simulink model "mclosed_loop_sim"  (Simulink 6.3)
settings: Solver=ode23s  SolverMode=SingleTasking  StartTime=0.0  StopTime=10  RelTol=1e-3  AbsTol=1e-6
PreLoadFcn:
  | Kp=0.0614;Ki=0.0723;
undefined symbols (not defined in the file or in its folder): DiscIntNeverNeededParam
settings Model: CovMetricSettings=d  Creator=The MathWorks Inc.  LastModifiedBy=mshakeri  ExtModeTrigMode=oneshot  ExtModeArmWhenConnect=off  ExtModeAutoUpdateStatusClock=off  StrictBusMsg=ErrorLevel1
settings DataIOCC: ExternalInput=[]  InitialState=[]  LimitDataPoints=off  SaveFormat=StructureWithTime  OutputSaveName=yout1
settings OptimizationCC: BooleanDataType=off  InlineParams=on  InlineInvariantSignals=on
settings DebuggingCC: CheckExecutionContextPreStartOutputMsg=on  CheckExecutionContextRuntimeOutputMsg=on  SolverPrmCheckMsg=none  IntegerOverflowMsg=none
settings HardwareCC: TargetUnknown=on

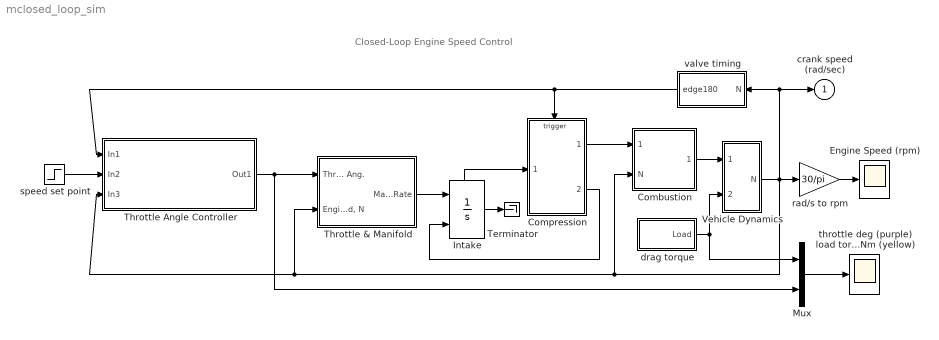
== system mclosed_loop_sim ==
  note: Closed-Loop Engine Speed Control
  Combustion : Subsystem
  Compression : Subsystem  TreatAsAtomicUnit=on
  Engine Speed (rpm) : Scope
      settings: TickLabels=on  YMin=1500  YMax=3500  SaveName=scopeout1
  Intake : Integrator  ExternalReset=either  ShowStatePort=on
  Mux : Mux  Inputs=2
  Terminator : Terminator
  Throttle & Manifold : Subsystem
  Throttle Angle Controller : Subsystem  TreatAsAtomicUnit=on
  Vehicle Dynamics : Subsystem
  drag torque : Subsystem
  rad/s to rpm : Gain  Gain=30/pi  SaturateOnIntegerOverflow=on
  speed set point : Step  Time=5  Before=2000  After=3000  SampleTime=0
  throttle deg (purple) load torque Nm (yellow) : Scope
      settings: TickLabels=on  YMin=5  YMax=30  SaveName=scopeout2
  valve timing : Subsystem  Orientation=left
  crank speed (rad/sec) : Outport  InitialOutput=0
  wires:
  speed set point/1 -> Throttle Angle Controller/2(In2)
  drag torque/1(Load) -> Mux/1, Vehicle Dynamics/2(Tload)
  Throttle Angle Controller/1(Out1) -> Throttle & Manifold/1(Throttle Ang.), Mux/2
  Compression/1(mass(k)) -> Combustion/1(Air Charge)
  Throttle & Manifold/1(Mass Airflow Rate) -> Intake/1
  Intake/1 -> Terminator/1
  Intake/State -> Compression/1(mass(k+1))
  Compression/2(trigger) -> Intake/2
  valve timing/1(edge180) -> Compression/Trigger, Throttle Angle Controller/1(In1)
  Combustion/1(Torque) -> Vehicle Dynamics/1(Teng)
  Vehicle Dynamics/1(N) -> Throttle & Manifold/2("Engine Speed, N"), Throttle Angle Controller/3(In3), Combustion/2(N), valve timing/1(N), crank speed (rad/sec)/1, rad/s to rpm/1
  rad/s to rpm/1 -> Engine Speed (rpm)/1
  Mux/1 -> throttle deg (purple) load torque Nm (yellow)/1

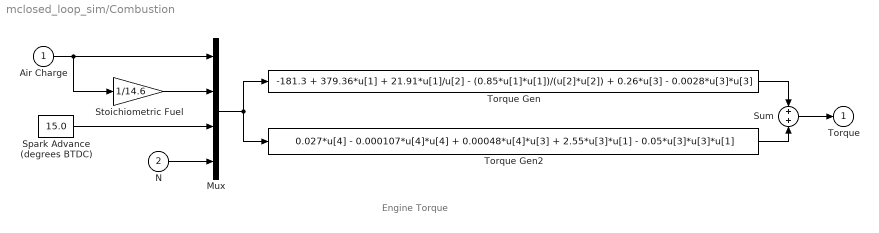
== system mclosed_loop_sim/Combustion ==
  note: Engine Torque
  Air Charge : Inport  Port=1  LatchInput=off
  N : Inport  Port=2  LatchInput=off
  Mux : Mux
  Spark Advance (degrees BTDC) : Constant  Value=15.0
  Stoichiometric Fuel : Gain  Gain=1/14.6  SaturateOnIntegerOverflow=on
  Sum : Sum  SaturateOnIntegerOverflow=on  InputSameDT=on
  Torque Gen : Fcn  Expr=-181.3 + 379.36*u[1] + 21.91*u[1]/u[2] - (0.85*u[1]*u[1])/(u[2]*u[2]) + 0.26*u[3] - 0.0028*u[3]*u[3]
  Torque Gen2 : Fcn  Expr=0.027*u[4] - 0.000107*u[4]*u[4] + 0.00048*u[4]*u[3] + 2.55*u[3]*u[1] - 0.05*u[3]*u[3]*u[1]
  Torque : Outport  InitialOutput=0
  wires:
  Stoichiometric Fuel/1 -> Mux/2
  Spark Advance (degrees BTDC)/1 -> Mux/3
  N/1 -> Mux/4
  Air Charge/1 -> Stoichiometric Fuel/1, Mux/1
  Mux/1 -> Torque Gen/1, Torque Gen2/1
  Torque Gen2/1 -> Sum/2
  Torque Gen/1 -> Sum/1
  Sum/1 -> Torque/1

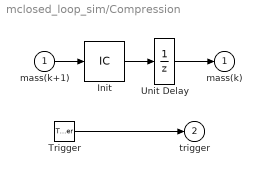
== system mclosed_loop_sim/Compression ==
  mass(k+1) : Inport  Port=1  LatchInput=off
  Trigger : TriggerPort  TriggerType=either  ShowOutputPort=on
  Init : InitialCondition  Value=0.152
  Unit Delay : UnitDelay  X0=0.152  SampleTime=-1
  mass(k) : Outport  InitialOutput=0.152
  trigger : Outport  Port=2  InitialOutput=-1
  wires:
  Init/1 -> Unit Delay/1
  mass(k+1)/1 -> Init/1
  Unit Delay/1 -> mass(k)/1
  Trigger/1 -> trigger/1

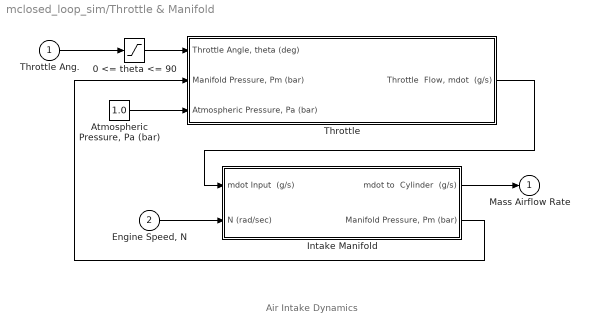
== system mclosed_loop_sim/Throttle & Manifold ==
  note: Air Intake Dynamics
  Throttle Ang. : Inport  Port=1  LatchInput=off
  "Engine Speed, N" : Inport  Port=2  LatchInput=off
  0 <= theta <= 90 : Saturate  UpperLimit=90  LowerLimit=0
  "Atmospheric Pressure, Pa (bar)" : Constant  Value=1.0
  Intake Manifold : Subsystem
  Throttle : Subsystem
  Mass Airflow Rate : Outport  InitialOutput=0
  wires:
  "Atmospheric Pressure, Pa (bar)"/1 -> Throttle/3("Atmospheric Pressure, Pa (bar) ")
  Intake Manifold/1(mdot to  Cylinder  (g/s)) -> Mass Airflow Rate/1
  Intake Manifold/2("Manifold Pressure, Pm (bar)") -> Throttle/2("Manifold Pressure, Pm (bar)")
  "Engine Speed, N"/1 -> Intake Manifold/2(N (rad/sec))
  Throttle/1("Throttle  Flow, mdot  (g/s)") -> Intake Manifold/1(mdot Input  (g/s))
  Throttle Ang./1 -> 0 <= theta <= 90/1
  0 <= theta <= 90/1 -> Throttle/1("Throttle Angle, theta (deg)")

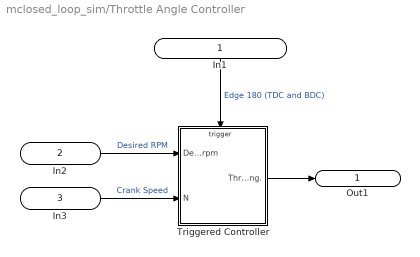
== system mclosed_loop_sim/Throttle Angle Controller ==
  In1 : Inport  Orientation=down  Port=1  LatchInput=off
  In2 : Inport  Port=2  SampleTime=[0 1]  LatchInput=off
  In3 : Inport  Port=3  SampleTime=[0 1]  LatchInput=off
  Triggered Controller : Subsystem  TreatAsAtomicUnit=on
  Out1 : Outport
  wires:
  In1/1 -> Triggered Controller/Trigger  "Edge 180 (TDC and BDC)"
  In3/1 -> Triggered Controller/2(N)  "Crank Speed"
  In2/1 -> Triggered Controller/1(Desired rpm)  "Desired RPM"
  Triggered Controller/1(Throttle Ang.) -> Out1/1

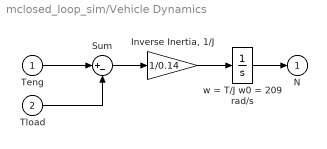
== system mclosed_loop_sim/Vehicle Dynamics ==
  Teng : Inport  Port=1  LatchInput=off
  Tload : Inport  Port=2  LatchInput=off
  "Inverse Inertia, 1/J" : Gain  Gain=1/0.14  SaturateOnIntegerOverflow=on
  Sum : Sum  Inputs=|+-  SaturateOnIntegerOverflow=on  InputSameDT=on
  w = T/J w0 = 209 rad/s : Integrator  InitialCondition=209.48
  N : Outport  InitialOutput=0
  wires:
  "Inverse Inertia, 1/J"/1 -> w = T/J w0 = 209 rad/s/1
  w = T/J w0 = 209 rad/s/1 -> N/1
  Sum/1 -> "Inverse Inertia, 1/J"/1
  Teng/1 -> Sum/1
  Tload/1 -> Sum/2

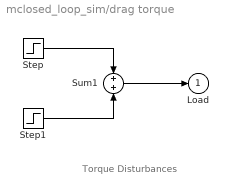
== system mclosed_loop_sim/drag torque ==
  note: Torque Disturbances
  Step : Step  Time=2  Before=25  After=20  SampleTime=0
  Step1 : Step  Time=8  After=5  SampleTime=0
  Sum1 : Sum  SaturateOnIntegerOverflow=on  InputSameDT=on
  Load : Outport  InitialOutput=0
  wires:
  Sum1/1 -> Load/1
  Step/1 -> Sum1/1
  Step1/1 -> Sum1/2

== system mclosed_loop_sim/valve timing ==
  note: Rotational Velocity to Synchronized
      | Discrete Event Conversion
  N : Inport  Orientation=left  Port=1  LatchInput=off
  TDC and BDC detection : Subsystem  Orientation=left
  positive edge to dual edge conversion : Subsystem  Orientation=left  TreatAsAtomicUnit=on
  edge180 : Outport  Orientation=left  InitialOutput=-1
  wires:
  TDC and BDC detection/1(trigger) -> positive edge to dual edge conversion/Trigger
  positive edge to dual edge conversion/1(trigger) -> edge180/1
  N/1 -> TDC and BDC detection/1(N)  "rad/sec"

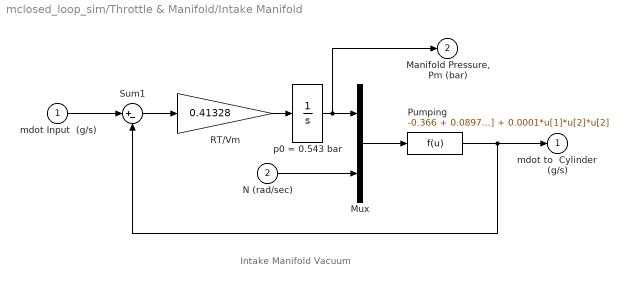
== system mclosed_loop_sim/Throttle & Manifold/Intake Manifold ==
  note: Intake Manifold Vacuum
  mdot Input  (g/s) : Inport  Port=1  LatchInput=off
  N (rad/sec) : Inport  Port=2  LatchInput=off
  Mux : Mux  Inputs=2
  Pumping : Fcn  Expr=-0.366 + 0.08979*u[1]*u[2] - 0.0337*u[2]*u[1]*u[1] + 0.0001*u[1]*u[2]*u[2]
  RT/Vm : Gain  Gain=0.41328  SaturateOnIntegerOverflow=on
  Sum1 : Sum  Inputs=|+-  SaturateOnIntegerOverflow=on  InputSameDT=on
  p0 = 0.543 bar : Integrator  InitialCondition=.543
  mdot to  Cylinder  (g/s) : Outport  InitialOutput=0
  "Manifold Pressure, Pm (bar)" : Outport  Port=2  InitialOutput=0
  wires:
  Pumping/1 -> mdot to  Cylinder  (g/s)/1, Sum1/2
  Sum1/1 -> RT/Vm/1
  p0 = 0.543 bar/1 -> "Manifold Pressure, Pm (bar)"/1, Mux/1
  Mux/1 -> Pumping/1
  N (rad/sec)/1 -> Mux/2
  RT/Vm/1 -> p0 = 0.543 bar/1
  mdot Input  (g/s)/1 -> Sum1/1

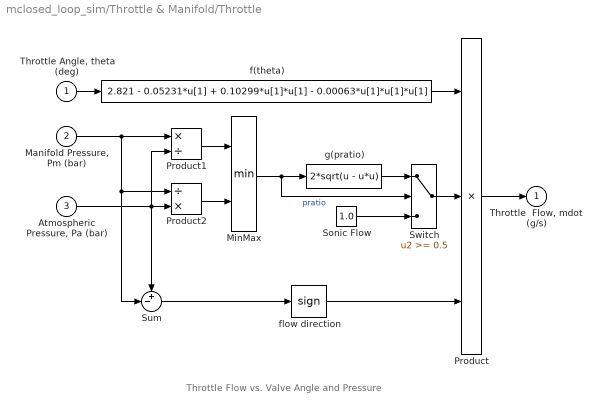
== system mclosed_loop_sim/Throttle & Manifold/Throttle ==
  note: Throttle Flow vs. Valve Angle and Pressure
  "Throttle Angle, theta (deg)" : Inport  Port=1  LatchInput=off
  "Manifold Pressure, Pm (bar)" : Inport  Port=2  LatchInput=off
  "Atmospheric Pressure, Pa (bar) " : Inport  Port=3  LatchInput=off
  MinMax : MinMax  Inputs=2  SaturateOnIntegerOverflow=on  InputSameDT=on
  Product : Product  Inputs=3  SaturateOnIntegerOverflow=on  RndMeth=Zero  InputSameDT=on
  Product1 : Product  Inputs=*/  SaturateOnIntegerOverflow=on  RndMeth=Zero  InputSameDT=on
  Product2 : Product  Inputs=/*  SaturateOnIntegerOverflow=on  RndMeth=Zero  InputSameDT=on
  "Sonic Flow " : Constant  Value=1.0
  Sum : Sum  Inputs=+-|  SaturateOnIntegerOverflow=on  InputSameDT=on
  Switch : Switch  Threshold=0.5  SaturateOnIntegerOverflow=on  InputSameDT=on
  f(theta) : Fcn  Expr=2.821 - 0.05231*u[1] + 0.10299*u[1]*u[1] - 0.00063*u[1]*u[1]*u[1]
  flow direction : Signum
  g(pratio) : Fcn  Expr=2*sqrt(u - u*u)
  "Throttle  Flow, mdot  (g/s)" : Outport  InitialOutput=0
  wires:
  f(theta)/1 -> Product/1
  Product/1 -> "Throttle  Flow, mdot  (g/s)"/1
  "Throttle Angle, theta (deg)"/1 -> f(theta)/1
  MinMax/1 -> g(pratio)/1, Switch/2  "pratio"
  Sum/1 -> flow direction/1
  flow direction/1 -> Product/3
  Switch/1 -> Product/2
  "Sonic Flow "/1 -> Switch/3
  g(pratio)/1 -> Switch/1
  "Atmospheric Pressure, Pa (bar) "/1 -> Product1/2, Product2/2, Sum/1
  Product1/1 -> MinMax/1
  Product2/1 -> MinMax/2
  "Manifold Pressure, Pm (bar)"/1 -> Product1/1, Product2/1, Sum/2

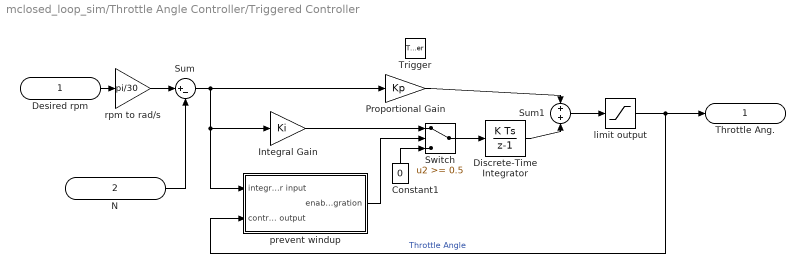
== system mclosed_loop_sim/Throttle Angle Controller/Triggered Controller ==
  Desired rpm : Inport  Port=1  LatchInput=off
  N : Inport  Port=2  LatchInput=off
  Trigger : TriggerPort  TriggerType=either
  Constant1 : Constant  Orientation=up  Value=0
  Discrete-Time Integrator : DiscreteIntegrator  InitialCondition=8.973  SampleTime=-1  ICPrevOutput=DiscIntNeverNeededParam  ICPrevScaledInput=DiscIntNeverNeededParam
  Integral Gain : Gain  Gain=Ki  SaturateOnIntegerOverflow=on
  Proportional Gain : Gain  Gain=Kp  SaturateOnIntegerOverflow=on
  Sum : Sum  Inputs=|+-  SaturateOnIntegerOverflow=on  InputSameDT=on
  Sum1 : Sum  SaturateOnIntegerOverflow=on  InputSameDT=on
  Switch : Switch  Threshold=0.5  SaturateOnIntegerOverflow=on  InputSameDT=on
  limit output : Saturate  UpperLimit=70  LowerLimit=0
  prevent windup : Subsystem
  rpm to rad/s : Gain  Gain=pi/30  SaturateOnIntegerOverflow=on
  Throttle Ang. : Outport  InitialOutput=8.973
  wires:
  rpm to rad/s/1 -> Sum/1
  Discrete-Time Integrator/1 -> Sum1/2
  limit output/1 -> prevent windup/2(controller output), Throttle Ang./1  "Throttle Angle"
  prevent windup/1(enable integration) -> Switch/2
  Sum1/1 -> limit output/1
  Switch/1 -> Discrete-Time Integrator/1
  Proportional Gain/1 -> Sum1/1
  Constant1/1 -> Switch/3
  Integral Gain/1 -> Switch/1
  Sum/1 -> prevent windup/1(integrator input), Integral Gain/1, Proportional Gain/1
  N/1 -> Sum/2
  Desired rpm/1 -> rpm to rad/s/1

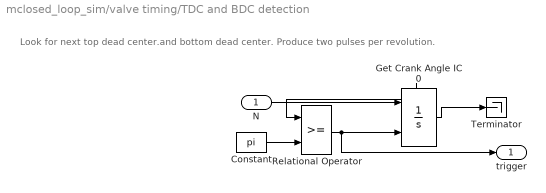
== system mclosed_loop_sim/valve timing/TDC and BDC detection ==
  note: Look for next top dead center.and
      | bottom dead center.
      | Produce two pulses per revolution.
  N : Inport  Port=1  LatchInput=off
  Constant : Constant  Value=pi
  Get Crank Angle IC 0 : Integrator  ExternalReset=rising  ShowStatePort=on
  Relational Operator : RelationalOperator  InputSameDT=on
  Terminator : Terminator
  trigger : Outport  InitialOutput=0
  wires:
  N/1 -> Get Crank Angle IC 0/1
  Relational Operator/1 -> trigger/1, Get Crank Angle IC 0/2
  Constant/1 -> Relational Operator/2
  Get Crank Angle IC 0/State -> Relational Operator/1
  Get Crank Angle IC 0/1 -> Terminator/1

== system mclosed_loop_sim/valve timing/positive edge to dual edge conversion ==
  Trigger : TriggerPort
  Gain : Gain  Orientation=left  Gain=-1  SaturateOnIntegerOverflow=on
  Unit Delay : UnitDelay  X0=1  SampleTime=-1
  trigger : Outport  InitialOutput=-1
  wires:
  Gain/1 -> Unit Delay/1
  Unit Delay/1 -> trigger/1, Gain/1

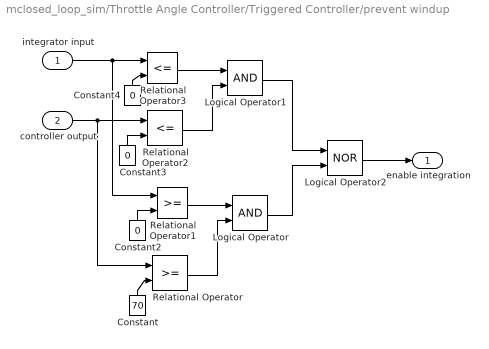
== system mclosed_loop_sim/Throttle Angle Controller/Triggered Controller/prevent windup ==
  integrator input : Inport  Port=1  LatchInput=off
  controller output : Inport  Port=2  LatchInput=off
  Constant : Constant  Orientation=up  Value=70
  Constant2 : Constant  Orientation=up  Value=0
  Constant3 : Constant  Orientation=up  Value=0
  Constant4 : Constant  Orientation=up  Value=0
  Logical Operator : Logic
  Logical Operator1 : Logic
  Logical Operator2 : Logic  Operator=NOR
  Relational Operator : RelationalOperator  InputSameDT=on
  Relational Operator1 : RelationalOperator  InputSameDT=on
  Relational Operator2 : RelationalOperator  Operator=<=  InputSameDT=on
  Relational Operator3 : RelationalOperator  Operator=<=  InputSameDT=on
  enable integration : Outport  InitialOutput=0
  wires:
  Logical Operator2/1 -> enable integration/1
  Logical Operator/1 -> Logical Operator2/2
  Logical Operator1/1 -> Logical Operator2/1
  Relational Operator/1 -> Logical Operator/2
  Relational Operator1/1 -> Logical Operator/1
  Constant/1 -> Relational Operator/2
  Constant2/1 -> Relational Operator1/2
  controller output/1 -> Relational Operator2/1, Relational Operator/1
  integrator input/1 -> Relational Operator3/1, Relational Operator1/1
  Relational Operator2/1 -> Logical Operator1/2
  Relational Operator3/1 -> Logical Operator1/1
  Constant4/1 -> Relational Operator3/2
  Constant3/1 -> Relational Operator2/2
